simulink model "Kinematic"  (R2019a)
settings: Solver=FixedStepAuto  StartTime=0.0  StopTime=200  FixedStep=0.01  RelTol=1e-3
settings Model: Creator=ADMIN  LastModifiedBy=ADMIN

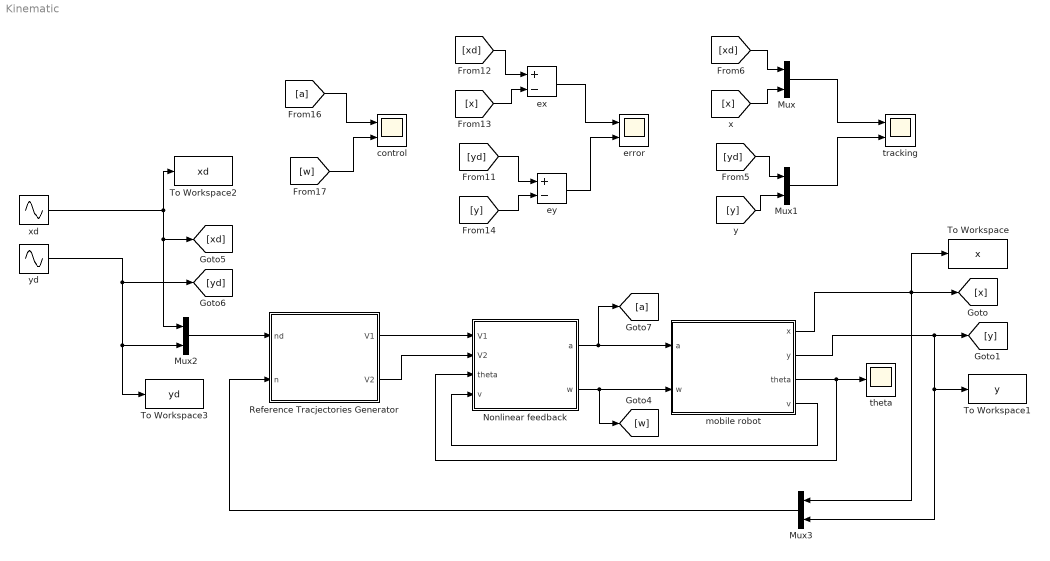
== system Kinematic ==
  Mux{,1..3} (4 alike) : Mux  Inputs=2
  Nonlinear feedback : Subsystem
  Reference Tracjectories Generator : Subsystem  mask{K2=10, K1=10}
      mask TypeOptions K2: KD1/Gain
      mask TypeOptions K1: KP1/Gain
  To Workspace : ToWorkspace  VariableName=x  SaveFormat=Timeseries  SampleTime=-1
  To Workspace1 : ToWorkspace  VariableName=y  SaveFormat=Timeseries  SampleTime=-1
  To Workspace2 : ToWorkspace  VariableName=xd  SaveFormat=Timeseries  SampleTime=-1
  To Workspace3 : ToWorkspace  VariableName=yd  SaveFormat=Timeseries  SampleTime=-1
  control : Scope  NumInputPorts=2
  error : Scope  NumInputPorts=2
  ex : Sum  Inputs=+-
  ey : Sum  Inputs=+-
  mobile robot : Subsystem  mask{x0=2, y0=3, theta0=0, v0=3}
      mask TypeOptions x0: Integrator/InitialCondition
      mask TypeOptions y0: Integrator1/InitialCondition
      mask TypeOptions theta0: Integrator2/InitialCondition
      mask TypeOptions v0: Integrator3/InitialCondition
  theta : Scope
  tracking : Scope  NumInputPorts=2
  xd : Sin  Amplitude=2  Frequency=0.05  Phase=pi/2  SampleTime=0
  yd : Sin  Amplitude=2  Frequency=0.05  SampleTime=0
  wires:
  Nonlinear feedback/1(a) -> [a], mobile robot/1(a)
  Reference Tracjectories Generator/1(V1) -> Nonlinear feedback/1(V1)
  Reference Tracjectories Generator/2(V2) -> Nonlinear feedback/2(V2)
  Nonlinear feedback/2(w) -> [w], mobile robot/2(w)
  Mux/1 -> tracking/1
  mobile robot/4(v) -> Nonlinear feedback/4(v)
  mobile robot/3(theta) -> theta/1, Nonlinear feedback/3(theta)
  mobile robot/1(x) -> Mux3/1, To Workspace/1, [x]
  mobile robot/2(y) -> Mux3/2, To Workspace1/1, [y]
  [xd] -> Mux/1
  [x] -> Mux/2
  Mux1/1 -> tracking/2
  [y] -> Mux1/2
  [yd] -> Mux1/1
  [x] -> ex/2
  [xd] -> ex/1
  [yd] -> ey/1
  [y] -> ey/2
  ex/1 -> error/1
  ey/1 -> error/2
  xd/1 -> Mux2/1, [xd], To Workspace2/1
  yd/1 -> [yd], Mux2/2, To Workspace3/1
  [a] -> control/1
  [w] -> control/2
  Mux2/1 -> Reference Tracjectories Generator/1(nd)
  Mux3/1 -> Reference Tracjectories Generator/2(n)

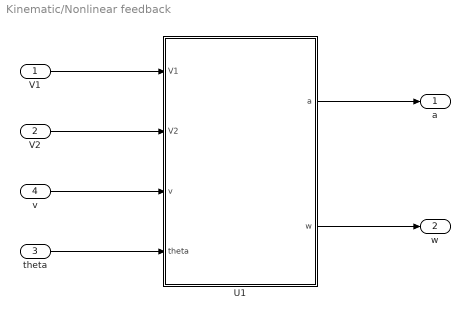
== system Kinematic/Nonlinear feedback ==
  V1 : Inport
  V2 : Inport  Port=2
  theta : Inport  Port=3
  v : Inport  Port=4
  U1 : MATLAB Function  TreatAsAtomicUnit=on
  a : Outport
  w : Outport  Port=2
  wires:
  V1/1 -> U1/1(V1)
  V2/1 -> U1/2(V2)
  U1/1(a) -> a/1
  U1/2(w) -> w/1
  theta/1 -> U1/4(theta)
  v/1 -> U1/3(v)

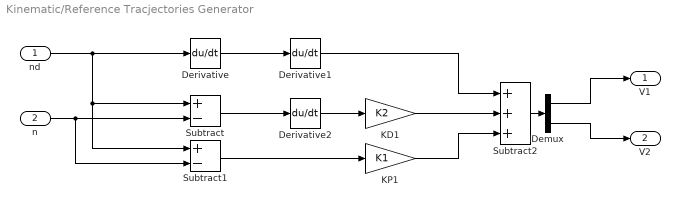
== system Kinematic/Reference Tracjectories Generator ==
  nd : Inport
  n : Inport  Port=2
  Demux : Demux  Outputs=2
  Derivative : Derivative
  Derivative1 : Derivative
  Derivative2 : Derivative
  KD1 : Gain  Gain=K2
  KP1 : Gain  Gain=K1
  Subtract : Sum  Inputs=+-
  Subtract1 : Sum  Inputs=+-
  Subtract2 : Sum  Inputs=+++
  V1 : Outport
  V2 : Outport  Port=2
  wires:
  Derivative/1 -> Derivative1/1
  Subtract/1 -> Derivative2/1
  Subtract1/1 -> KP1/1
  Derivative1/1 -> Subtract2/1
  KP1/1 -> Subtract2/3
  n/1 -> Subtract1/2, Subtract/2
  nd/1 -> Subtract1/1, Subtract/1, Derivative/1
  Derivative2/1 -> KD1/1
  KD1/1 -> Subtract2/2
  Demux/2 -> V2/1
  Subtract2/1 -> Demux/1
  Demux/1 -> V1/1

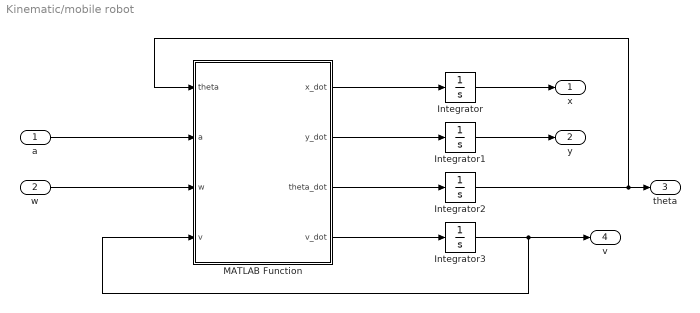
== system Kinematic/mobile robot ==
  a : Inport
  w : Inport  Port=2
  Integrator : Integrator  InitialCondition=x0
  Integrator1 : Integrator  InitialCondition=y0
  Integrator2 : Integrator  InitialCondition=theta0
  Integrator3 : Integrator  InitialCondition=v0
  MATLAB Function : MATLAB Function  TreatAsAtomicUnit=on
  x : Outport
  y : Outport  Port=2
  theta : Outport  Port=3
  v : Outport  Port=4
  wires:
  Integrator/1 -> x/1
  Integrator1/1 -> y/1
  Integrator2/1 -> theta/1, MATLAB Function/1(theta)
  Integrator3/1 -> v/1, MATLAB Function/4(v)
  a/1 -> MATLAB Function/2(a)
  w/1 -> MATLAB Function/3(w)
  MATLAB Function/1(x_dot) -> Integrator/1
  MATLAB Function/2(y_dot) -> Integrator1/1
  MATLAB Function/3(theta_dot) -> Integrator2/1
  MATLAB Function/4(v_dot) -> Integrator3/1

== matlab function Kinematic/Nonlinear feedback/U1 ==
  data: V1 input; a output; V2 input; v input; theta input; w output
function [a,w] = fcn(V1, V2, v, theta)
a = V1*cos(theta) + V2*sin(theta);
w = (V2*cos(theta) - V1*sin(theta))/v;

== matlab function Kinematic/mobile robot/MATLAB Function ==
  data: theta input; a input; x_dot output; w input; y_dot output; theta_dot output; v_dot output; v input
function [x_dot,y_dot,theta_dot,v_dot] = fcn(theta, a, w, v)
x_dot = v*cos(theta);
y_dot = v*sin(theta);
theta_dot = w;
v_dot = a;
end
